simulink model "sim_traj_output"  (R2025b)
settings: Solver=VariableStepAuto  StartTime=0.0  StopTime=10.0  RelTol=1e-3
undefined symbols (not defined in the file): Ts
settings Model: Creator=noyan  LastModifiedBy=noyan

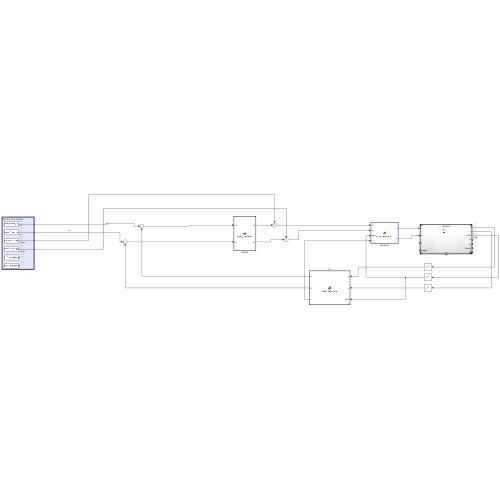
[thumbnail: Simulink's stored preview of the top-level diagram]
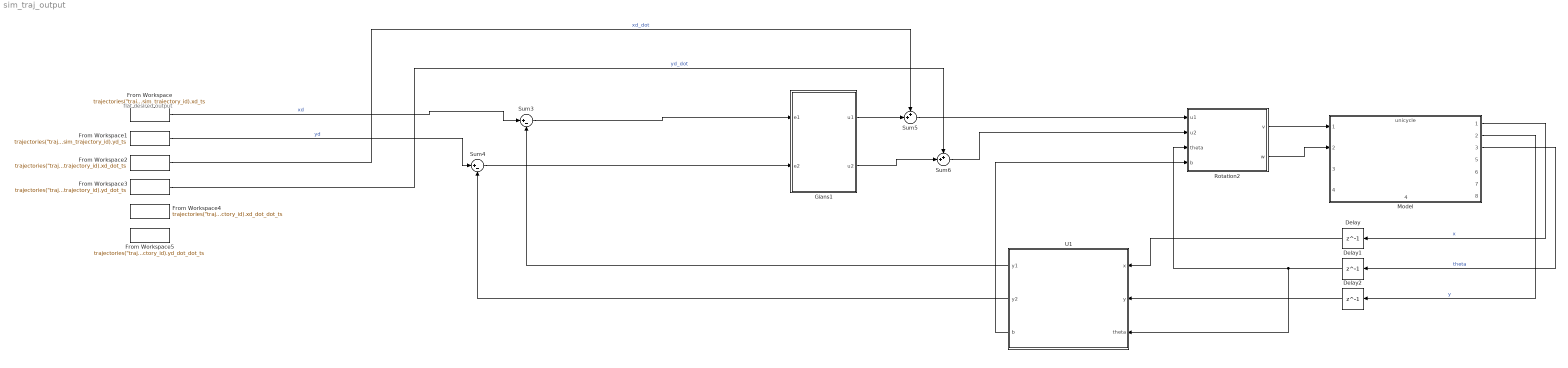
== system sim_traj_output ==
  note: flat desired output
  Delay : Delay  DelayLength=1
  Delay1 : Delay  DelayLength=1
  Delay2 : Delay  DelayLength=1
  From Workspace : FromWorkspace  VariableName="trajectories(\"trajectory\"+sim_trajectory_id).xd_ts"  SampleTime=Ts  OutputAfterFinalValue=Holding final value
  From Workspace1 : FromWorkspace  VariableName="trajectories(\"trajectory\"+sim_trajectory_id).yd_ts"  SampleTime=Ts  OutputAfterFinalValue=Holding final value
  From Workspace2 : FromWorkspace  VariableName="trajectories(\"trajectory\"+sim_trajectory_id).xd_dot_ts"  SampleTime=Ts  OutputAfterFinalValue=Holding final value
  From Workspace3 : FromWorkspace  VariableName="trajectories(\"trajectory\"+sim_trajectory_id).yd_dot_ts"  SampleTime=Ts  OutputAfterFinalValue=Holding final value
  From Workspace4 : FromWorkspace  VariableName="trajectories(\"trajectory\"+sim_trajectory_id).xd_dot_dot_ts"  SampleTime=Ts  OutputAfterFinalValue=Holding final value
  From Workspace5 : FromWorkspace  VariableName="trajectories(\"trajectory\"+sim_trajectory_id).yd_dot_dot_ts"  SampleTime=Ts  OutputAfterFinalValue=Holding final value
  Gians1 : MATLAB Function  TreatAsAtomicUnit=on
  Model : ModelReference  ModelNameDialog=unicycle.slx  SimulationMode=Normal  ModelReferenceVersion=1.12
      settings: PortSchema="{\"entries\":[{\"content\":{\"sides\":[{\"content\":{\"connectorIds\":[\"In1\",\"In2\",\"In3\",\"In4\"]},\"type\":\"ConnectorPlacement.EquallySpacedRectSide\",\"uuid\":\"ad25d81c-9301-4260-b0e7-6964e2a4144d\"},{\"content\":{\"connectorIds\":[\"Out1\",\"Out2\",\"Out3\",\"Out5\",\"Out6\",\"Out7\",\"Out8\"],\"side\":\"RIGHT\"},\"type\":\"ConnectorPlacement.EquallySpacedRectSide\",\"uuid\":\"e119e278-1a19-4d21-ac57-f30b4b2846c4\"},{\"content\":{\"side\":\"TOP\"},\"type\":\"ConnectorPlacement.EquallySpacedRectSide\",\"uuid\":\"f58ebd06-2844-4b35-9f44-2944c544d228\"},{\"content\":{\"connectorIds\":[\"Out4\"],\"side\":\"BOTTOM\"},\"type\":\"ConnectorPlacement.EquallySpacedRectSide\",\"uuid\":\"e9666c6b-2f60-424a-96df-bac3fd1a20e8\"}]},\"type\":\"ConnectorPlacement.EquallySpacedConnector\",\"uuid\":\"feeb8aec-4c5e-4f88-9f0a-836c4fc89b7c\"}],\"packageUris\":[\"http://schema.mathworks.com/mf0/Connector/R2020b\"],\"version\":\"1.0\"}"
  Rotation2 : MATLAB Function  TreatAsAtomicUnit=on
  Sum3 : Sum  Inputs=|+-
  Sum4 : Sum  Inputs=|+-
  Sum5 : Sum  Inputs=++|
  Sum6 : Sum  Inputs=++|
  U1 : MATLAB Function  TreatAsAtomicUnit=on
  wires:
  Gians1/1(u1) -> Sum5/2
  U1/3(b) -> Rotation2/4(b)
  Sum4/1 -> Gians1/2(e2)
  Gians1/2(u2) -> Sum6/2
  U1/2(y2) -> Sum4/2
  Rotation2/2(w) -> Model/2
  Sum6/1 -> Rotation2/2(u2)
  Rotation2/1(v) -> Model/1
  Sum5/1 -> Rotation2/1(u1)
  Sum3/1 -> Gians1/1(e1)
  U1/1(y1) -> Sum3/2
  Model/3 -> Delay1/1  "theta"
  Model/1 -> Delay/1  "x"
  Model/2 -> Delay2/1  "y"
  From Workspace/1 -> Sum3/1  "xd"
  From Workspace2/1 -> Sum5/1  "xd_dot"
  From Workspace3/1 -> Sum6/1  "yd_dot"
  From Workspace1/1 -> Sum4/1  "yd"
  Delay/1 -> U1/1(x)
  Delay1/1 -> Rotation2/3(theta), U1/3(theta)
  Delay2/1 -> U1/2(y)

== matlab function sim_traj_output/Rotation2 ==
  data: u1 input; v output; u2 input; theta input; w output; b input
function [v,w] = error_transform(u1, u2 , theta,b)

v = u1 * cos(theta)       + u2 * sin(theta);
w = u1 * (- sin(theta)/b) + u2 *cos(theta)/b;
end

== matlab function sim_traj_output/Gians1 ==
  data: e1 input; u1 output; u2 output; e2 input
function [u1,u2 ] = gain_scheduler(e1,e2)

k1 = 1.5;
k2 = 1.5;

u1 = k1 * e1;
u2 = k2 * e2;



end

== matlab function sim_traj_output/U1 ==
  data: x input; y input; theta input; y1 output; y2 output; b output
function [y1, y2,b] = inversTransform(x,y,theta)
b = 1;
y1 = x + b * cos(theta);
y2 = y + b * sin(theta);

end
